simulink model "DiscretePID"  (R2021a)
settings: Solver=ode45  StartTime=0.0  StopTime=1.5  FixedStep=T_samp  RelTol=1e-4
undefined symbols (not defined in the file): AW, back, daq, DiscIntNeverNeededParam, drv, est_par, gbox, mot, pid, rads2rpm, rpm2degs, sens, simp_model, T_samp, tust
libraries: simulink x2
settings Model: Creator=Utente  LastModifiedBy=gioel
settings SolverCC: AlgebraicLoopSolver=TrustRegion
settings DataIOCC: ReturnWorkspaceOutputs=off
settings DebuggingCC: AlgebraicLoopMsg=none  SFMachineParentedDataDiag=warning

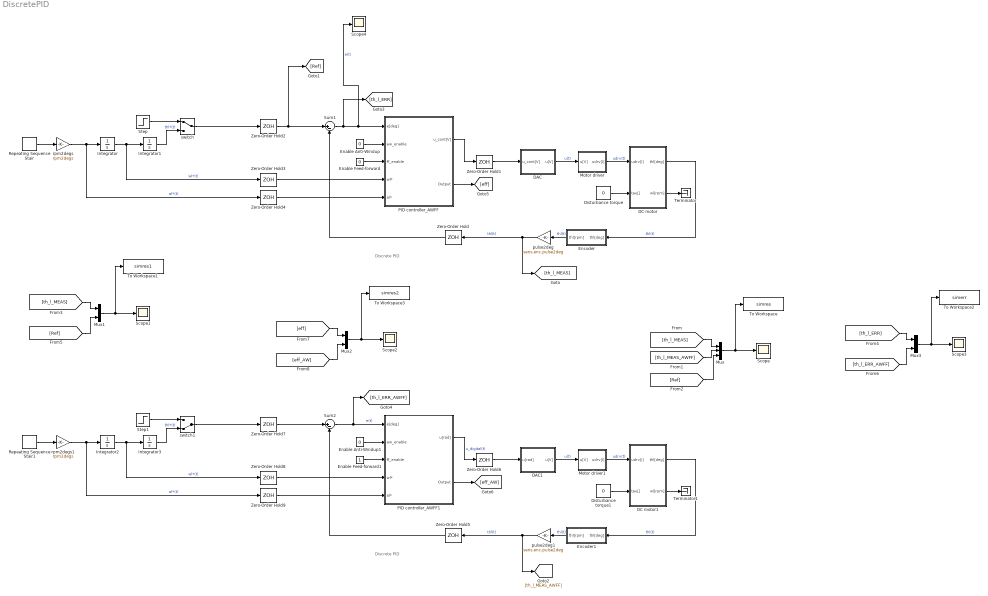
== system DiscretePID ==
  note: Discrete PID
  note: Discrete PID
  DAC : Subsystem
  DAC1 : Subsystem
  DC motor : Subsystem
  DC motor1 : Subsystem
  Disturbance torque : Constant  Value=0
  Disturbance torque1 : Constant  Value=0
  Enable Anti-Windup : Constant  Value=0
  Enable Anti-Windup1 : Constant  Value=0
  Enable Feed-forward : Constant  Value=0
  Enable Feed-forward1 : Constant
  Encoder : Subsystem
  Encoder1 : Subsystem
  Integrator{,1..3} (4 alike) : Integrator
  Motor driver : Subsystem
  Motor driver1 : Subsystem
  Mux : Mux  Inputs=3
  Mux1 : Mux  Inputs=2
  Mux2 : Mux  Inputs=2
  Mux3 : Mux  Inputs=2
  PID controller_AWFF : Subsystem
  PID controller_AWFF1 : Subsystem
  Repeating Sequence Stair : simulink/Sources/Repeating Sequence Stair  OutValues=[900 0 -900 -900 0 900].'  tsamp=0.5  OutMin=[]  OutMax=[]  OutDataTypeStr=double  OutputDataTypeScalingMode=double  OutDataType=fixdt(0,8)  ConRadixGroup=Best Precision: Vector-wise  OutScaling=2^-12
  Repeating Sequence Stair1 : simulink/Sources/Repeating Sequence Stair  OutValues=[900 0 -900 -900 0 900].'  tsamp=0.5  OutMin=[]  OutMax=[]  OutDataTypeStr=double  OutputDataTypeScalingMode=double  OutDataType=fixdt(0,8)  ConRadixGroup=Best Precision: Vector-wise  OutScaling=2^-12
  Scope{,1..4} (5 alike) : Scope
  Step : Step  Time=0  After=50  SampleTime=0
  Step1 : Step  Time=0  After=360  SampleTime=0
  Sum1 : Sum  Inputs=|+-
  Sum2 : Sum  Inputs=|+-
  Terminator : Terminator
  Terminator1 : Terminator
  To Workspace : ToWorkspace  VariableName=simres  SaveFormat=Structure With Time  SampleTime=-1
  To Workspace1 : ToWorkspace  VariableName=simres1  SaveFormat=Structure With Time  SampleTime=-1
  To Workspace2 : ToWorkspace  VariableName=simerr  SaveFormat=Structure With Time  SampleTime=-1
  To Workspace3 : ToWorkspace  VariableName=simres2  SaveFormat=Structure With Time  SampleTime=-1
  Zero-Order Hold{,1..9} (10 alike) : ZeroOrderHold  SampleTime=T_samp
  pulse2deg : Gain  Gain=sens.enc.pulse2deg
  pulse2deg1 : Gain  Gain=sens.enc.pulse2deg
  rpm2degs : Gain  Gain=rpm2degs
  rpm2degs1 : Gain  Gain=rpm2degs
  switch : ManualSwitch
  switch1 : ManualSwitch  CurrentSetting=0
  wires:
  DC motor/1(thl[deg]) -> Encoder/1(thl[deg])  "thl(t)"
  DAC/1(u[V]) -> Motor driver/1(u[V])  "u(t)"
  pulse2deg/1 -> Zero-Order Hold/1, [th_l_MEAS]  "thl(t)"
  Motor driver/1(udrv[I]) -> DC motor/1(udrv[I])  "udrv(t)"
  Encoder/1(thl[rpm]) -> pulse2deg/1  "thl(t)"
  Disturbance torque/1 -> DC motor/2(tau[])
  DC motor/2(wl[rpm]) -> Terminator/1
  Zero-Order Hold1/1 -> DAC/1(u_cont[V])
  Zero-Order Hold/1 -> Sum1/2
  Zero-Order Hold2/1 -> Sum1/1, [Ref]
  [th_l_MEAS] -> Mux/1
  [th_l_MEAS_AWFF] -> Mux/2
  Mux/1 -> To Workspace/1, Scope/1
  Enable Anti-Windup/1 -> PID controller_AWFF/2(aw_enable)
  Enable Feed-forward/1 -> PID controller_AWFF/3(ff_enable)
  PID controller_AWFF/1(u_cont[V]) -> Zero-Order Hold1/1
  Sum1/1 -> Scope4/1, PID controller_AWFF/1(e[deg]), [th_l_ERR]  "e(t)"
  Repeating Sequence Stair/1 -> rpm2degs/1
  Integrator1/1 -> switch/2  "thl*(t)"
  rpm2degs/1 -> Zero-Order Hold4/1, Integrator/1  "al*(t)"
  Integrator/1 -> Zero-Order Hold3/1, Integrator1/1  "wl*(t)"
  switch/1 -> Zero-Order Hold2/1
  Step/1 -> switch/1
  Zero-Order Hold3/1 -> PID controller_AWFF/4(wl*)
  Zero-Order Hold4/1 -> PID controller_AWFF/5(al*)
  Zero-Order Hold5/1 -> Sum2/2
  Repeating Sequence Stair1/1 -> rpm2degs1/1
  pulse2deg1/1 -> Zero-Order Hold5/1, [th_l_MEAS_AWFF]  "thl(t)"
  Zero-Order Hold8/1 -> PID controller_AWFF1/4(wl*)
  Enable Feed-forward1/1 -> PID controller_AWFF1/3(ff_enable)
  Encoder1/1(thl[rpm]) -> pulse2deg1/1  "thl(t)"
  rpm2degs1/1 -> Zero-Order Hold9/1, Integrator2/1  "al*(t)"
  DAC1/1(u[V]) -> Motor driver1/1(u[V])  "u(t)"
  Zero-Order Hold7/1 -> Sum2/1
  Motor driver1/1(udrv[I]) -> DC motor1/1(udrv[I])  "udrv(t)"
  switch1/1 -> Zero-Order Hold7/1
  Zero-Order Hold6/1 -> DAC1/1(u[rad])
  Step1/1 -> switch1/1
  Zero-Order Hold9/1 -> PID controller_AWFF1/5(al*)
  DC motor1/1(thl[deg]) -> Encoder1/1(thl[deg])  "thl(t)"
  Enable Anti-Windup1/1 -> PID controller_AWFF1/2(aw_enable)
  Integrator3/1 -> switch1/2  "thl*(t)"
  DC motor1/2(wl[rpm]) -> Terminator1/1
  Disturbance torque1/1 -> DC motor1/2(tau[])
  Integrator2/1 -> Zero-Order Hold8/1, Integrator3/1  "wl*(t)"
  PID controller_AWFF1/1(u[rad]) -> Zero-Order Hold6/1  "u_digital(t)"
  Sum2/1 -> [th_l_ERR_AWFF], PID controller_AWFF1/1(e[deg])  "e(t)"
  [Ref] -> Mux/3
  Mux1/1 -> Scope1/1, To Workspace1/1
  [th_l_MEAS] -> Mux1/1
  [Ref] -> Mux1/2
  [th_l_ERR_AWFF] -> Mux3/2
  Mux3/1 -> Scope3/1, To Workspace2/1
  [th_l_ERR] -> Mux3/1
  [eff_AW] -> Mux2/2
  Mux2/1 -> Scope2/1, To Workspace3/1
  [eff] -> Mux2/1
  PID controller_AWFF/2(Output) -> [eff]
  PID controller_AWFF1/2(Output) -> [eff_AW]

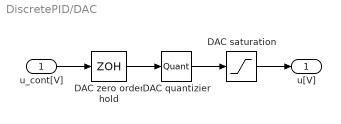
== system DiscretePID/DAC ==
  u_cont[V] : Inport
  DAC quantizier : Quantizer  QuantizationInterval=daq.dac.q
  DAC saturation : Saturate  UpperLimit=10  LowerLimit=-10
  DAC zero order hold : ZeroOrderHold  SampleTime=sens.enc.T_s
  u[V] : Outport
  wires:
  DAC quantizier/1 -> DAC saturation/1
  DAC zero order hold/1 -> DAC quantizier/1
  DAC saturation/1 -> u[V]/1
  u_cont[V]/1 -> DAC zero order hold/1

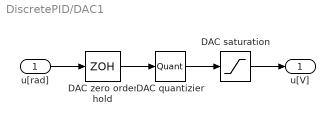
== system DiscretePID/DAC1 ==
  u[rad] : Inport
  DAC quantizier : Quantizer  QuantizationInterval=daq.dac.q
  DAC saturation : Saturate  UpperLimit=10  LowerLimit=-10
  DAC zero order hold : ZeroOrderHold  SampleTime=sens.enc.T_s
  u[V] : Outport
  wires:
  DAC quantizier/1 -> DAC saturation/1
  DAC zero order hold/1 -> DAC quantizier/1
  DAC saturation/1 -> u[V]/1
  u[rad]/1 -> DAC zero order hold/1

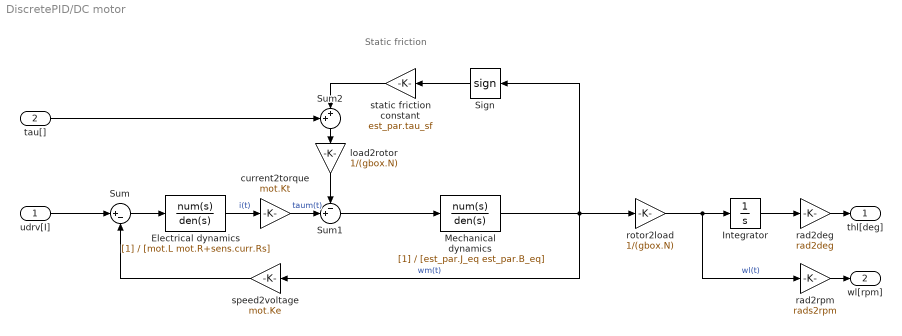
== system DiscretePID/DC motor ==
  note: Static friction
  udrv[I] : Inport  Unit=V
  tau[] : Inport  Port=2  Unit=V
  Electrical dynamics : TransferFcn  Denominator=[mot.L mot.R+sens.curr.Rs]
  Integrator : Integrator
  Mechanical dynamics : TransferFcn  Denominator=[est_par.J_eq est_par.B_eq]
  Sign : Signum  ZeroCross=off
  Sum : Sum  Inputs=|+-
  Sum1 : Sum  Inputs=-+|
  Sum2 : Sum  Inputs=++|
  current2torque : Gain  Gain=mot.Kt
  load2rotor : Gain  Gain=1/(gbox.N)
  rad2deg : Gain  Gain=rad2deg
  rad2rpm : Gain  Gain=rads2rpm
  rotor2load : Gain  Gain=1/(gbox.N)
  speed2voltage : Gain  Gain=mot.Ke
  static friction constant : Gain  Gain=est_par.tau_sf
  thl[deg] : Outport  Unit=deg
  wl[rpm] : Outport  Port=2  Unit=rpm
  wires:
  load2rotor/1 -> Sum1/1
  Mechanical dynamics/1 -> Sign/1, rotor2load/1, speed2voltage/1  "wm(t)"
  Sign/1 -> static friction constant/1
  current2torque/1 -> Sum1/2  "taum(t)"
  Sum1/1 -> Mechanical dynamics/1
  speed2voltage/1 -> Sum/2
  rotor2load/1 -> rad2rpm/1, Integrator/1  "wl(t)"
  Electrical dynamics/1 -> current2torque/1  "i(t)"
  Integrator/1 -> rad2deg/1
  Sum/1 -> Electrical dynamics/1
  rad2rpm/1 -> wl[rpm]/1
  rad2deg/1 -> thl[deg]/1
  udrv[I]/1 -> Sum/1
  static friction constant/1 -> Sum2/2
  Sum2/1 -> load2rotor/1
  tau[]/1 -> Sum2/1

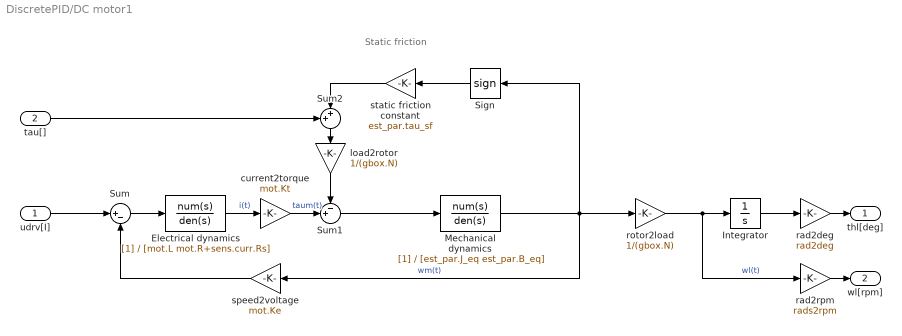
== system DiscretePID/DC motor1 ==
  note: Static friction
  udrv[I] : Inport  Unit=V
  tau[] : Inport  Port=2  Unit=V
  Electrical dynamics : TransferFcn  Denominator=[mot.L mot.R+sens.curr.Rs]
  Integrator : Integrator
  Mechanical dynamics : TransferFcn  Denominator=[est_par.J_eq est_par.B_eq]
  Sign : Signum  ZeroCross=off
  Sum : Sum  Inputs=|+-
  Sum1 : Sum  Inputs=-+|
  Sum2 : Sum  Inputs=++|
  current2torque : Gain  Gain=mot.Kt
  load2rotor : Gain  Gain=1/(gbox.N)
  rad2deg : Gain  Gain=rad2deg
  rad2rpm : Gain  Gain=rads2rpm
  rotor2load : Gain  Gain=1/(gbox.N)
  speed2voltage : Gain  Gain=mot.Ke
  static friction constant : Gain  Gain=est_par.tau_sf
  thl[deg] : Outport  Unit=deg
  wl[rpm] : Outport  Port=2  Unit=rpm
  wires:
  load2rotor/1 -> Sum1/1
  Mechanical dynamics/1 -> Sign/1, rotor2load/1, speed2voltage/1  "wm(t)"
  Sign/1 -> static friction constant/1
  current2torque/1 -> Sum1/2  "taum(t)"
  Sum1/1 -> Mechanical dynamics/1
  speed2voltage/1 -> Sum/2
  rotor2load/1 -> rad2rpm/1, Integrator/1  "wl(t)"
  Electrical dynamics/1 -> current2torque/1  "i(t)"
  Integrator/1 -> rad2deg/1
  Sum/1 -> Electrical dynamics/1
  rad2rpm/1 -> wl[rpm]/1
  rad2deg/1 -> thl[deg]/1
  udrv[I]/1 -> Sum/1
  static friction constant/1 -> Sum2/2
  Sum2/1 -> load2rotor/1
  tau[]/1 -> Sum2/1

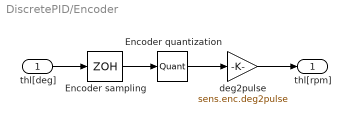
== system DiscretePID/Encoder ==
  thl[deg] : Inport
  Encoder quantization : Quantizer  QuantizationInterval=sens.enc.q
  Encoder sampling : ZeroOrderHold  SampleTime=sens.enc.T_s
  deg2pulse : Gain  Gain=sens.enc.deg2pulse
  thl[rpm] : Outport
  wires:
  Encoder quantization/1 -> deg2pulse/1
  deg2pulse/1 -> thl[rpm]/1
  Encoder sampling/1 -> Encoder quantization/1
  thl[deg]/1 -> Encoder sampling/1

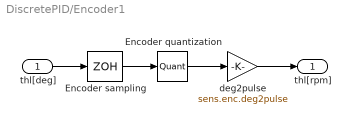
== system DiscretePID/Encoder1 ==
  thl[deg] : Inport
  Encoder quantization : Quantizer  QuantizationInterval=sens.enc.q
  Encoder sampling : ZeroOrderHold  SampleTime=sens.enc.T_s
  deg2pulse : Gain  Gain=sens.enc.deg2pulse
  thl[rpm] : Outport
  wires:
  Encoder quantization/1 -> deg2pulse/1
  deg2pulse/1 -> thl[rpm]/1
  Encoder sampling/1 -> Encoder quantization/1
  thl[deg]/1 -> Encoder sampling/1

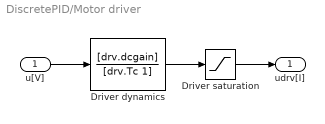
== system DiscretePID/Motor driver ==
  u[V] : Inport
  Driver dynamics : TransferFcn  Numerator=[drv.dcgain]  Denominator=[drv.Tc 1]
  Driver saturation : Saturate  UpperLimit=12  LowerLimit=-12
  udrv[I] : Outport
  wires:
  Driver saturation/1 -> udrv[I]/1
  Driver dynamics/1 -> Driver saturation/1
  u[V]/1 -> Driver dynamics/1

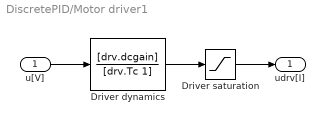
== system DiscretePID/Motor driver1 ==
  u[V] : Inport
  Driver dynamics : TransferFcn  Numerator=[drv.dcgain]  Denominator=[drv.Tc 1]
  Driver saturation : Saturate  UpperLimit=12  LowerLimit=-12
  udrv[I] : Outport
  wires:
  Driver saturation/1 -> udrv[I]/1
  Driver dynamics/1 -> Driver saturation/1
  u[V]/1 -> Driver dynamics/1

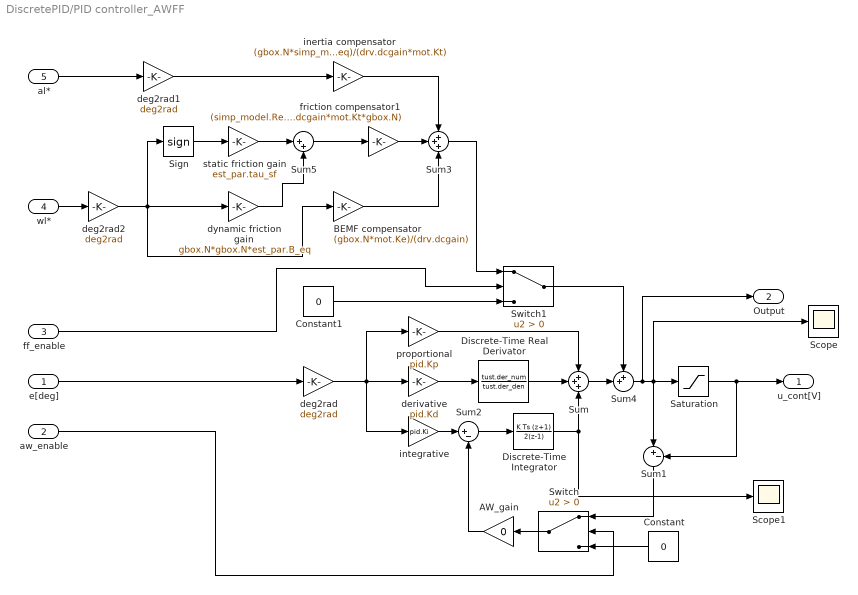
== system DiscretePID/PID controller_AWFF ==
  e[deg] : Inport  Unit=deg
  aw_enable : Inport  Port=2  Unit=deg
  ff_enable : Inport  Port=3  Unit=deg
  wl* : Inport  Port=4  Unit=deg
  al* : Inport  Port=5  Unit=deg
  AW_gain : Gain  Gain=0
  BEMF compensator : Gain  Gain=(gbox.N*mot.Ke)/(drv.dcgain)
  Constant : Constant  Value=0
  Constant1 : Constant  Value=0
  Discrete-Time Integrator : DiscreteIntegrator  IntegratorMethod=Integration: Trapezoidal  SampleTime=T_samp  ICPrevOutput=DiscIntNeverNeededParam  ICPrevScaledInput=DiscIntNeverNeededParam
  Discrete-Time Real Derivator : DiscreteTransferFcn  Numerator=tust.der_num  Denominator=tust.der_den  SampleTime=T_samp
  Saturation : Saturate  UpperLimit=daq.dac.vdd  LowerLimit=daq.dac.vss
  Scope : Scope
  Scope1 : Scope
  Sign : Signum
  Sum : Sum  Inputs=+++
  Sum1 : Sum  Inputs=|+-
  Sum2 : Sum  Inputs=|+-
  Sum3 : Sum  Inputs=+++
  Sum4 : Sum  Inputs=++|
  Sum5 : Sum  Inputs=|++
  Switch : Switch  Criteria=u2 > Threshold
  Switch1 : Switch  Criteria=u2 > Threshold
  deg2rad : Gain  Gain=deg2rad
  deg2rad1 : Gain  Gain=deg2rad
  deg2rad2 : Gain  Gain=deg2rad
  derivative : Gain  Gain=pid.Kd
  dynamic friction gain : Gain  Gain=gbox.N*gbox.N*est_par.B_eq
  friction compensator1 : Gain  Gain=(simp_model.Req)/(drv.dcgain*mot.Kt*gbox.N)
  inertia compensator : Gain  Gain=(gbox.N*simp_model.Req*est_par.J_eq)/(drv.dcgain*mot.Kt)
  integrative : Gain  Gain=pid.Ki
  proportional : Gain  Gain=pid.Kp
  static friction gain : Gain  Gain=est_par.tau_sf
  u_cont[V] : Outport
  Output : Outport  Port=2
  wires:
  e[deg]/1 -> deg2rad/1
  deg2rad/1 -> integrative/1, derivative/1, proportional/1
  proportional/1 -> Sum/1
  Saturation/1 -> Sum1/2, u_cont[V]/1
  integrative/1 -> Sum2/1
  Sum2/1 -> Discrete-Time Integrator/1
  AW_gain/1 -> Sum2/2
  Discrete-Time Real Derivator/1 -> Sum/2
  derivative/1 -> Discrete-Time Real Derivator/1
  aw_enable/1 -> Switch/2
  Constant/1 -> Switch/3
  Switch/1 -> AW_gain/1
  Sum1/1 -> Switch/1
  ff_enable/1 -> Switch1/2
  Constant1/1 -> Switch1/3
  friction compensator1/1 -> Sum3/2
  inertia compensator/1 -> Sum3/1
  BEMF compensator/1 -> Sum3/3
  Sum4/1 -> Output/1, Scope/1, Saturation/1, Sum1/1
  Sign/1 -> static friction gain/1
  static friction gain/1 -> Sum5/1
  dynamic friction gain/1 -> Sum5/2
  Sum5/1 -> friction compensator1/1
  al*/1 -> deg2rad1/1
  wl*/1 -> deg2rad2/1
  Sum3/1 -> Switch1/1
  Sum/1 -> Sum4/2
  deg2rad1/1 -> inertia compensator/1
  deg2rad2/1 -> BEMF compensator/1, Sign/1, dynamic friction gain/1
  Discrete-Time Integrator/1 -> Sum/3, Scope1/1
  Switch1/1 -> Sum4/1

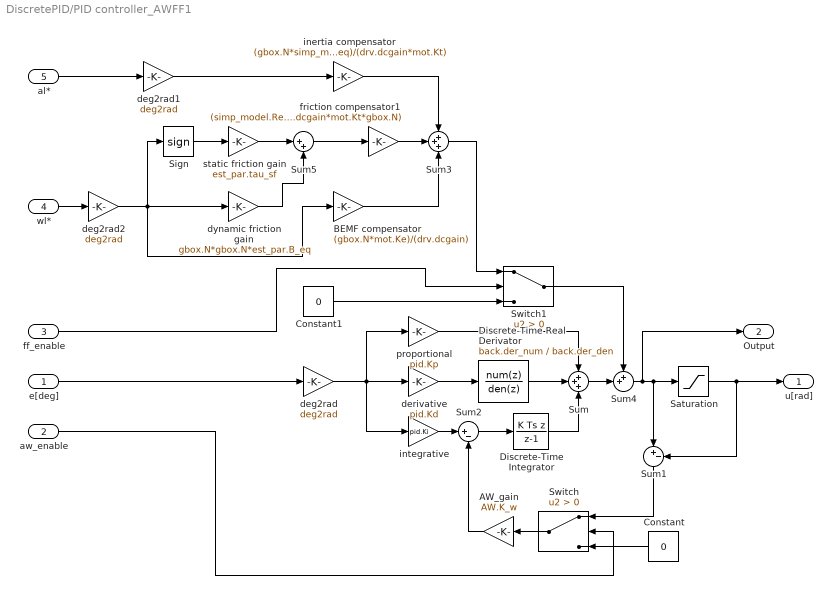
== system DiscretePID/PID controller_AWFF1 ==
  e[deg] : Inport  Unit=deg
  aw_enable : Inport  Port=2  Unit=deg
  ff_enable : Inport  Port=3  Unit=deg
  wl* : Inport  Port=4  Unit=deg
  al* : Inport  Port=5  Unit=deg
  AW_gain : Gain  Gain=AW.K_w
  BEMF compensator : Gain  Gain=(gbox.N*mot.Ke)/(drv.dcgain)
  Constant : Constant  Value=0
  Constant1 : Constant  Value=0
  Discrete-Time Integrator : DiscreteIntegrator  IntegratorMethod=Integration: Backward Euler  SampleTime=T_samp  ICPrevOutput=DiscIntNeverNeededParam  ICPrevScaledInput=DiscIntNeverNeededParam
  Discrete-Time Real Derivator : DiscreteTransferFcn  Numerator=back.der_num  Denominator=back.der_den  SampleTime=T_samp
  Saturation : Saturate  UpperLimit=daq.dac.vdd  LowerLimit=daq.dac.vss
  Sign : Signum
  Sum : Sum  Inputs=+++
  Sum1 : Sum  Inputs=|+-
  Sum2 : Sum  Inputs=|+-
  Sum3 : Sum  Inputs=+++
  Sum4 : Sum  Inputs=++|
  Sum5 : Sum  Inputs=|++
  Switch : Switch  Criteria=u2 > Threshold
  Switch1 : Switch  Criteria=u2 > Threshold
  deg2rad : Gain  Gain=deg2rad
  deg2rad1 : Gain  Gain=deg2rad
  deg2rad2 : Gain  Gain=deg2rad
  derivative : Gain  Gain=pid.Kd
  dynamic friction gain : Gain  Gain=gbox.N*gbox.N*est_par.B_eq
  friction compensator1 : Gain  Gain=(simp_model.Req)/(drv.dcgain*mot.Kt*gbox.N)
  inertia compensator : Gain  Gain=(gbox.N*simp_model.Req*est_par.J_eq)/(drv.dcgain*mot.Kt)
  integrative : Gain  Gain=pid.Ki
  proportional : Gain  Gain=pid.Kp
  static friction gain : Gain  Gain=est_par.tau_sf
  u[rad] : Outport
  Output : Outport  Port=2
  wires:
  e[deg]/1 -> deg2rad/1
  deg2rad/1 -> integrative/1, derivative/1, proportional/1
  proportional/1 -> Sum/1
  Saturation/1 -> Sum1/2, u[rad]/1
  integrative/1 -> Sum2/1
  Sum2/1 -> Discrete-Time Integrator/1
  AW_gain/1 -> Sum2/2
  Discrete-Time Real Derivator/1 -> Sum/2
  derivative/1 -> Discrete-Time Real Derivator/1
  aw_enable/1 -> Switch/2
  Constant/1 -> Switch/3
  Switch/1 -> AW_gain/1
  Sum1/1 -> Switch/1
  ff_enable/1 -> Switch1/2
  Constant1/1 -> Switch1/3
  friction compensator1/1 -> Sum3/2
  inertia compensator/1 -> Sum3/1
  BEMF compensator/1 -> Sum3/3
  Sum4/1 -> Output/1, Saturation/1, Sum1/1
  Sign/1 -> static friction gain/1
  static friction gain/1 -> Sum5/1
  dynamic friction gain/1 -> Sum5/2
  Sum5/1 -> friction compensator1/1
  al*/1 -> deg2rad1/1
  wl*/1 -> deg2rad2/1
  Sum3/1 -> Switch1/1
  Sum/1 -> Sum4/2
  deg2rad1/1 -> inertia compensator/1
  deg2rad2/1 -> BEMF compensator/1, Sign/1, dynamic friction gain/1
  Discrete-Time Integrator/1 -> Sum/3
  Switch1/1 -> Sum4/1
